simulink model "m01_PMSM_Desktop"  (R2023b)
settings: Solver=FixedStepAuto  StartTime=0.0  StopTime=0.6  FixedStep=Ts  RelTol=1e-3  AbsTol=1e-3
PreLoadFcn:
  | control_data;
  | pmsm_data;
undefined symbols (not defined in the file): avgFactor, Gs, J, Tmax, Ts, Tsc
libraries: fl_lib x54, nesl_utility x53, ee_lib x13, SimscapeFPGAHIL_lib x12, eePmsmFieldOrientedControl x1
(part 2 of 2)

== system m01_PMSM_Desktop/Inverter/Pejovic w//SCA/Switch4 ==
  G : Inport
  Controller : SimscapeFPGAHIL_lib/Linearized Switch Models/Switch/Controller  threshold=threshold  Gs=Gs  s=timeScaling  avgFactor=avgFactor  isFixedPoint=off
  Gs : fl_lib/Electrical/Electrical Elements/Resistor  R=1/Gs Ohm  i_specify=off  i_priority=None  i=0 A  i_nominal_specify=off  i_nominal_unit=A  i_nominal_value=1  v_specify=off  v_priority=None  v=0 V  v_nominal_specify=off  v_nominal_unit=V  v_nominal_value=1
      settings: LibrarySourceBlock=SimscapeFPGAHIL_lib/Linearized Switch Models/Switch/Gs
  ic : fl_lib/Electrical/Electrical Sources/Controlled Current Source
      settings: LibrarySourceBlock=SimscapeFPGAHIL_lib/Linearized Switch Models/Switch/ic
  ic_in : nesl_utility/Simulink-PS Converter  PhysicalDomain=network_engine_domain  SubClassName=ps_input  LeftPortType=input  RightPortType=output  PseudoPeriodic=off  Frequencies=[]  NoiseDistribution=none  NoiseParameters=[]  Unit=A  AffineConversion=off  FilteringAndDerivatives=provide  SimscapeFilterOrder=1  InputFilterTimeConstant=0.001  UdotUserProvided=0
      settings: LibrarySourceBlock=SimscapeFPGAHIL_lib/Linearized Switch Models/Switch/ic_in
  is : fl_lib/Electrical/Electrical Sensors/Current Sensor
      settings: LibrarySourceBlock=SimscapeFPGAHIL_lib/Linearized Switch Models/Switch/is
  is_out : nesl_utility/PS-Simulink Converter  PhysicalDomain=network_engine_domain  SubClassName=ps_output  LeftPortType=input  RightPortType=output  PseudoPeriodic=off  Frequencies=[]  VectorFormat=1-D array  Unit=A  AffineConversion=off
      settings: LibrarySourceBlock=SimscapeFPGAHIL_lib/Linearized Switch Models/Switch/is_out
  vs : fl_lib/Electrical/Electrical Sensors/Voltage Sensor
      settings: LibrarySourceBlock=SimscapeFPGAHIL_lib/Linearized Switch Models/Switch/vs
  vs_out : nesl_utility/PS-Simulink Converter  PhysicalDomain=network_engine_domain  SubClassName=ps_output  LeftPortType=input  RightPortType=output  PseudoPeriodic=off  Frequencies=[]  VectorFormat=1-D array  Unit=V  AffineConversion=off
      settings: LibrarySourceBlock=SimscapeFPGAHIL_lib/Linearized Switch Models/Switch/vs_out
  + : PMIOPort  Side=Left
  - : PMIOPort  Port=2  Side=Right
  wires:
  Controller/1 -> ic_in/1
  G/1 -> Controller/3
  is_out/1 -> Controller/2
  vs_out/1 -> Controller/1
  connections:
  is_out/LConn1 -- is/RConn1
  vs_out/LConn1 -- vs/RConn1
  ic_in/RConn1 -- ic/RConn1
  is/LConn1 -- +/RConn1 -- vs/LConn1
  ic/RConn2 -- Gs/RConn1 -- -/RConn1 -- vs/RConn2
  is/RConn2 -- Gs/LConn1 -- ic/LConn1

== system m01_PMSM_Desktop/Inverter/Pejovic w//SCA/Switch5 ==
  G : Inport
  Controller : SimscapeFPGAHIL_lib/Linearized Switch Models/Switch/Controller  threshold=threshold  Gs=Gs  s=timeScaling  avgFactor=avgFactor  isFixedPoint=off
  Gs : fl_lib/Electrical/Electrical Elements/Resistor  R=1/Gs Ohm  i_specify=off  i_priority=None  i=0 A  i_nominal_specify=off  i_nominal_unit=A  i_nominal_value=1  v_specify=off  v_priority=None  v=0 V  v_nominal_specify=off  v_nominal_unit=V  v_nominal_value=1
      settings: LibrarySourceBlock=SimscapeFPGAHIL_lib/Linearized Switch Models/Switch/Gs
  ic : fl_lib/Electrical/Electrical Sources/Controlled Current Source
      settings: LibrarySourceBlock=SimscapeFPGAHIL_lib/Linearized Switch Models/Switch/ic
  ic_in : nesl_utility/Simulink-PS Converter  PhysicalDomain=network_engine_domain  SubClassName=ps_input  LeftPortType=input  RightPortType=output  PseudoPeriodic=off  Frequencies=[]  NoiseDistribution=none  NoiseParameters=[]  Unit=A  AffineConversion=off  FilteringAndDerivatives=provide  SimscapeFilterOrder=1  InputFilterTimeConstant=0.001  UdotUserProvided=0
      settings: LibrarySourceBlock=SimscapeFPGAHIL_lib/Linearized Switch Models/Switch/ic_in
  is : fl_lib/Electrical/Electrical Sensors/Current Sensor
      settings: LibrarySourceBlock=SimscapeFPGAHIL_lib/Linearized Switch Models/Switch/is
  is_out : nesl_utility/PS-Simulink Converter  PhysicalDomain=network_engine_domain  SubClassName=ps_output  LeftPortType=input  RightPortType=output  PseudoPeriodic=off  Frequencies=[]  VectorFormat=1-D array  Unit=A  AffineConversion=off
      settings: LibrarySourceBlock=SimscapeFPGAHIL_lib/Linearized Switch Models/Switch/is_out
  vs : fl_lib/Electrical/Electrical Sensors/Voltage Sensor
      settings: LibrarySourceBlock=SimscapeFPGAHIL_lib/Linearized Switch Models/Switch/vs
  vs_out : nesl_utility/PS-Simulink Converter  PhysicalDomain=network_engine_domain  SubClassName=ps_output  LeftPortType=input  RightPortType=output  PseudoPeriodic=off  Frequencies=[]  VectorFormat=1-D array  Unit=V  AffineConversion=off
      settings: LibrarySourceBlock=SimscapeFPGAHIL_lib/Linearized Switch Models/Switch/vs_out
  + : PMIOPort  Side=Left
  - : PMIOPort  Port=2  Side=Right
  wires:
  vs_out/1 -> Controller/1
  is_out/1 -> Controller/2
  G/1 -> Controller/3
  Controller/1 -> ic_in/1
  connections:
  ic/LConn1 -- Gs/LConn1 -- is/RConn2
  vs/RConn2 -- -/RConn1 -- Gs/RConn1 -- ic/RConn2
  vs/LConn1 -- +/RConn1 -- is/LConn1
  ic_in/RConn1 -- ic/RConn1
  vs_out/LConn1 -- vs/RConn1
  is_out/LConn1 -- is/RConn1

== system m01_PMSM_Desktop/Inverter/Pejovic w//SCA/Switch6 ==
  G : Inport
  Controller : SimscapeFPGAHIL_lib/Linearized Switch Models/Switch/Controller  threshold=threshold  Gs=Gs  s=timeScaling  avgFactor=avgFactor  isFixedPoint=off
  Gs : fl_lib/Electrical/Electrical Elements/Resistor  R=1/Gs Ohm  i_specify=off  i_priority=None  i=0 A  i_nominal_specify=off  i_nominal_unit=A  i_nominal_value=1  v_specify=off  v_priority=None  v=0 V  v_nominal_specify=off  v_nominal_unit=V  v_nominal_value=1
      settings: LibrarySourceBlock=SimscapeFPGAHIL_lib/Linearized Switch Models/Switch/Gs
  ic : fl_lib/Electrical/Electrical Sources/Controlled Current Source
      settings: LibrarySourceBlock=SimscapeFPGAHIL_lib/Linearized Switch Models/Switch/ic
  ic_in : nesl_utility/Simulink-PS Converter  PhysicalDomain=network_engine_domain  SubClassName=ps_input  LeftPortType=input  RightPortType=output  PseudoPeriodic=off  Frequencies=[]  NoiseDistribution=none  NoiseParameters=[]  Unit=A  AffineConversion=off  FilteringAndDerivatives=provide  SimscapeFilterOrder=1  InputFilterTimeConstant=0.001  UdotUserProvided=0
      settings: LibrarySourceBlock=SimscapeFPGAHIL_lib/Linearized Switch Models/Switch/ic_in
  is : fl_lib/Electrical/Electrical Sensors/Current Sensor
      settings: LibrarySourceBlock=SimscapeFPGAHIL_lib/Linearized Switch Models/Switch/is
  is_out : nesl_utility/PS-Simulink Converter  PhysicalDomain=network_engine_domain  SubClassName=ps_output  LeftPortType=input  RightPortType=output  PseudoPeriodic=off  Frequencies=[]  VectorFormat=1-D array  Unit=A  AffineConversion=off
      settings: LibrarySourceBlock=SimscapeFPGAHIL_lib/Linearized Switch Models/Switch/is_out
  vs : fl_lib/Electrical/Electrical Sensors/Voltage Sensor
      settings: LibrarySourceBlock=SimscapeFPGAHIL_lib/Linearized Switch Models/Switch/vs
  vs_out : nesl_utility/PS-Simulink Converter  PhysicalDomain=network_engine_domain  SubClassName=ps_output  LeftPortType=input  RightPortType=output  PseudoPeriodic=off  Frequencies=[]  VectorFormat=1-D array  Unit=V  AffineConversion=off
      settings: LibrarySourceBlock=SimscapeFPGAHIL_lib/Linearized Switch Models/Switch/vs_out
  + : PMIOPort  Side=Left
  - : PMIOPort  Port=2  Side=Right
  wires:
  Controller/1 -> ic_in/1
  G/1 -> Controller/3
  is_out/1 -> Controller/2
  vs_out/1 -> Controller/1
  connections:
  is_out/LConn1 -- is/RConn1
  vs_out/LConn1 -- vs/RConn1
  ic_in/RConn1 -- ic/RConn1
  is/LConn1 -- +/RConn1 -- vs/LConn1
  ic/RConn2 -- Gs/RConn1 -- -/RConn1 -- vs/RConn2
  is/RConn2 -- Gs/LConn1 -- ic/LConn1

== system m01_PMSM_Desktop/Inverter/Simscape Converter/Gates ==
  Gates Simulink : Inport
  Demux : Demux  Outputs=6
  GaH : nesl_utility/Simulink-PS Converter  PhysicalDomain=network_engine_domain  SubClassName=ps_input  LeftPortType=input  RightPortType=output  PseudoPeriodic=off  Frequencies=[]  NoiseDistribution=none  NoiseParameters=[]  Unit=1  AffineConversion=off  FilteringAndDerivatives=zero  SimscapeFilterOrder=1  InputFilterTimeConstant=0.001  UdotUserProvided=0
  GaL : nesl_utility/Simulink-PS Converter  PhysicalDomain=network_engine_domain  SubClassName=ps_input  LeftPortType=input  RightPortType=output  PseudoPeriodic=off  Frequencies=[]  NoiseDistribution=none  NoiseParameters=[]  Unit=1  AffineConversion=off  FilteringAndDerivatives=zero  SimscapeFilterOrder=1  InputFilterTimeConstant=0.001  UdotUserProvided=0
  GbH : nesl_utility/Simulink-PS Converter  PhysicalDomain=network_engine_domain  SubClassName=ps_input  LeftPortType=input  RightPortType=output  PseudoPeriodic=off  Frequencies=[]  NoiseDistribution=none  NoiseParameters=[]  Unit=1  AffineConversion=off  FilteringAndDerivatives=zero  SimscapeFilterOrder=1  InputFilterTimeConstant=0.001  UdotUserProvided=0
  GbL : nesl_utility/Simulink-PS Converter  PhysicalDomain=network_engine_domain  SubClassName=ps_input  LeftPortType=input  RightPortType=output  PseudoPeriodic=off  Frequencies=[]  NoiseDistribution=none  NoiseParameters=[]  Unit=1  AffineConversion=off  FilteringAndDerivatives=zero  SimscapeFilterOrder=1  InputFilterTimeConstant=0.001  UdotUserProvided=0
  GcH : nesl_utility/Simulink-PS Converter  PhysicalDomain=network_engine_domain  SubClassName=ps_input  LeftPortType=input  RightPortType=output  PseudoPeriodic=off  Frequencies=[]  NoiseDistribution=none  NoiseParameters=[]  Unit=1  AffineConversion=off  FilteringAndDerivatives=zero  SimscapeFilterOrder=1  InputFilterTimeConstant=0.001  UdotUserProvided=0
  GcL : nesl_utility/Simulink-PS Converter  PhysicalDomain=network_engine_domain  SubClassName=ps_input  LeftPortType=input  RightPortType=output  PseudoPeriodic=off  Frequencies=[]  NoiseDistribution=none  NoiseParameters=[]  Unit=1  AffineConversion=off  FilteringAndDerivatives=zero  SimscapeFilterOrder=1  InputFilterTimeConstant=0.001  UdotUserProvided=0
  Six-Pulse Gate Multiplexer : ee_lib/Semiconductors & Converters/Converters/Six-Pulse Gate Multiplexer  port_option=ee.enum.controlport.ps
  Gates PS : PMIOPort  Side=Right
  wires:
  Demux/6 -> GcL/1
  Demux/3 -> GbH/1
  Demux/1 -> GaH/1
  Demux/4 -> GbL/1
  Demux/2 -> GaL/1
  Gates Simulink/1 -> Demux/1
  Demux/5 -> GcH/1
  connections:
  Six-Pulse Gate Multiplexer/LConn4 -- GbL/RConn1
  Six-Pulse Gate Multiplexer/LConn5 -- GcH/RConn1
  GaL/RConn1 -- Six-Pulse Gate Multiplexer/LConn2
  GaH/RConn1 -- Six-Pulse Gate Multiplexer/LConn1
  Six-Pulse Gate Multiplexer/LConn6 -- GcL/RConn1
  Six-Pulse Gate Multiplexer/LConn3 -- GbH/RConn1
  Six-Pulse Gate Multiplexer/RConn1 -- Gates PS/RConn1
